simulink model "Lab2Quanser"  (R2021b)
settings: Solver=ode1  StartTime=0.0  StopTime=10  FixedStep=Ts  RelTol=1e-3
InitFcn:
  | Ts=1e-3;
undefined symbols (not defined in the file): Model_626, Sensoray
libraries: sldrtlib x2
settings Model: SimulationMode=external  ExtModeTrigDuration=10001  Creator=Melab1Guest  LastModifiedBy=Melab1Guest
settings RTWCC: Description=Simulink Desktop Real-Time  SystemTargetFile=sldrt.tlc  TemplateMakefile=sldrt.tmf  RTWCompilerOptimization=on
settings CodeAppCC: MaxIdLength=95
settings SimulinkDesktopRealTimeCC: TargetPreCompLibLocation=C:\Program Files\MATLAB\R2021b\toolbox\sldrt\lib\win64

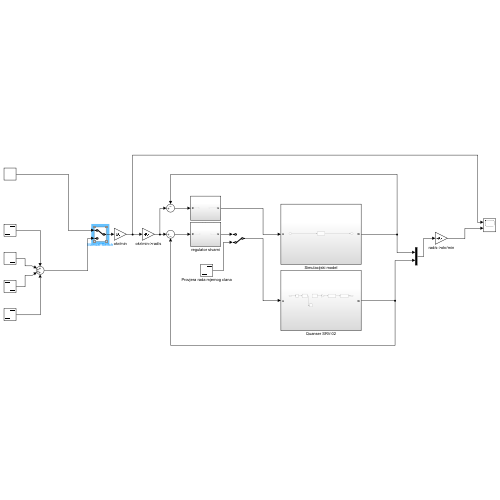
[thumbnail: Simulink's stored preview of the top-level diagram]
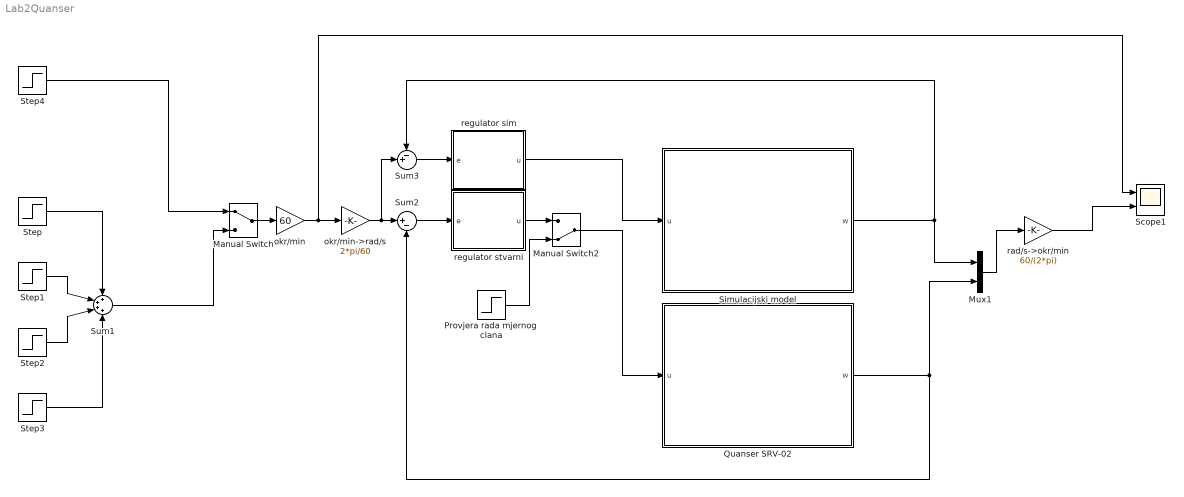
== system Lab2Quanser ==
  Manual Switch : ManualSwitch
  Manual Switch2 : ManualSwitch  CurrentSetting=0
  Mux1 : Mux  Inputs=2
  Provjera rada mjernog clana : Step  Time=2  After=3  SampleTime=0
  Quanser SRV-02 : Subsystem
  Scope1 : Scope  NumInputPorts=2
  Simulacijski model : Subsystem
  Step : Step  Time=2  SampleTime=0
  Step1 : Step  Time=4  After=-1  SampleTime=0
  Step2 : Step  Time=6  After=-1  SampleTime=0
  Step3 : Step  Time=8  SampleTime=0
  Step4 : Step  Time=2  SampleTime=0
  Sum1 : Sum  Inputs=++++
  Sum2 : Sum  Inputs=|+-
  Sum3 : Sum  Inputs=-+|
  okr/min : Gain  Gain=60
  okr/min->rad/s : Gain  Gain=2*pi/60
  rad/s->okr/min : Gain  Gain=60/(2*pi)
  regulator sim : Subsystem
  regulator stvarni : Subsystem
  wires:
  Sum2/1 -> regulator stvarni/1(e)
  Step/1 -> Sum1/1
  Step1/1 -> Sum1/2
  Step2/1 -> Sum1/3
  Step3/1 -> Sum1/4
  Manual Switch/1 -> okr/min/1
  Step4/1 -> Manual Switch/1
  Sum1/1 -> Manual Switch/2
  okr/min/1 -> Scope1/1, okr/min->rad/s/1
  okr/min->rad/s/1 -> Sum3/2, Sum2/1
  Simulacijski model/1(w) -> Sum3/1, Mux1/1
  rad/s->okr/min/1 -> Scope1/2
  regulator stvarni/1(u) -> Manual Switch2/1
  Provjera rada mjernog clana/1 -> Manual Switch2/2
  Sum3/1 -> regulator sim/1(e)
  regulator sim/1(u) -> Simulacijski model/1(u)
  Manual Switch2/1 -> Quanser SRV-02/1(u)
  Quanser SRV-02/1(w) -> Mux1/2, Sum2/2
  Mux1/1 -> rad/s->okr/min/1

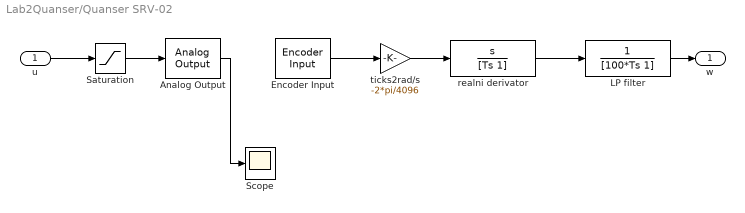
== system Lab2Quanser/Quanser SRV-02 ==
  u : Inport
  Analog Output : sldrtlib/Analog Output  SampleTime=Ts  MaxMissedTicks=100  ShowMissedTicks=on  YieldWhenWaiting=off  DrvName=Sensoray/Model_626  DrvAddress=4294967295  DrvOptions=zeros(1,0)  Channels=1  RangeMode=1  VoltRange=1  InitialValue=0  FinalValue=0
      settings: AttributesFormatString=Sensoray\nModel 626 [auto]
  Encoder Input : sldrtlib/Encoder Input  SampleTime=Ts  MaxMissedTicks=100  ShowMissedTicks=off  YieldWhenWaiting=off  DrvName=Sensoray/Model_626  DrvAddress=4294967295  DrvOptions=zeros(1,0)  Channels=1  QuadMode=3  IndexPulse=2  InputFilter=Inf  DataType=1
      settings: AttributesFormatString=Sensoray\nModel 626 [auto]
  LP filter : TransferFcn  Denominator=[100*Ts 1]
  Saturation : Saturate  UpperLimit=6  LowerLimit=-6
  Scope : Scope
  realni derivator : TransferFcn  Numerator=[1 0]  Denominator=[Ts 1]
  ticks2rad/s : Gain  Gain=-2*pi/4096
  w : Outport
  wires:
  Encoder Input/1 -> ticks2rad/s/1
  ticks2rad/s/1 -> realni derivator/1
  Analog Output/1 -> Scope/1
  realni derivator/1 -> LP filter/1
  LP filter/1 -> w/1
  u/1 -> Saturation/1
  Saturation/1 -> Analog Output/1

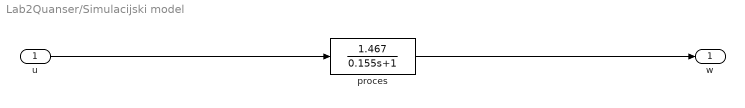
== system Lab2Quanser/Simulacijski model ==
  u : Inport
  proces : TransferFcn  Numerator=[1.467]  Denominator=[0.155 1]
  w : Outport
  wires:
  proces/1 -> w/1
  u/1 -> proces/1

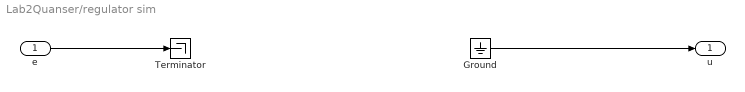
== system Lab2Quanser/regulator sim ==
  e : Inport
  Ground : Ground
  Terminator : Terminator
  u : Outport
  wires:
  Ground/1 -> u/1
  e/1 -> Terminator/1

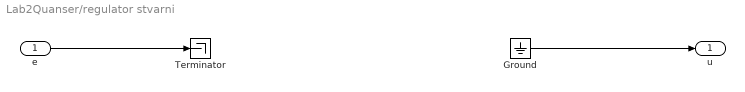
== system Lab2Quanser/regulator stvarni ==
  e : Inport
  Ground : Ground
  Terminator : Terminator
  u : Outport
  wires:
  e/1 -> Terminator/1
  Ground/1 -> u/1
